simulink model "GlobalMessageLevel_R2010b"  (Simulink 7.6)
settings: Solver=ode45  StartTime=0.0  StopTime=10.0  RelTol=1e-3
undefined symbols (not defined in the file): Carnot_density_Callbacks, Carnot_GlobalMessageLevel_Callbacks
settings Model: DEBUGGLOBALLEVEL=DEBUG  DEBUGMAXTOTALWARNINGS=inf  DEBUGMAXCONSECUTIVEWARNINGS=inf  DEBUGWRITETOFILE=0  DEBUGFILENAME='error.txt'  Creator=awohlfei  LastModifiedBy=awohlfei
settings OptimizationCC: ExpressionDepthLimit=128
settings DebuggingCC: FcnCallInpInsideContextMsg=Enable All
settings CodeAppCC: CustomSymbolStrType=$N$R$M_T

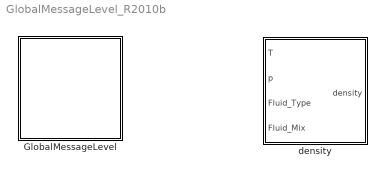
== system GlobalMessageLevel_R2010b ==
  GlobalMessageLevel : Subsystem  LoadFcn=Carnot_GlobalMessageLevel_Callbacks('LoadFcn');  mask(Global Message Level){GLOBALLOCAL=global, DEBUGLEVEL=DEBUG, MAXTOTALWARNINGS=inf, MAXCONSECUTIVEWARNINGS=inf, WRITETOFILE=0, FILENAME='error.txt'}
      mask prompts: GLOBALLOCAL "message settings"; DEBUGLEVEL "message level"; MAXTOTALWARNINGS "maximum total number of warnings"; MAXCONSECUTIVEWARNINGS "maxmum consecutive warnings"; WRITETOFILE "write messages to file"
      mask help: This block sets the message level of the complete model.
      mask init:
      | Carnot_GlobalMessageLevel_Callbacks('SetData');
      mask StyleString: popup(global|local),popup(DEBUG|INFO|WARNING|ERROR|FATAL|NONE),edit,edit,edit,edit
      mask CallbackString: Carnot_GlobalMessageLevel_Callbacks('MaskCallback');|||||
      mask Display:
      | fprintf(get_param(gcb, 'GLOBALLOCAL'));
      | fprintf(['\n\n', get_param(gcb, 'DEBUGLEVEL')]);
  density : Subsystem  LoadFcn=Carnot_density_Callbacks('LoadFcn');  InitFcn=load('THB.mat');  mask(density){INPUTARGUMENTS=state variables (classic), DEBUGLEVEL=DEBUG, MAXTOTALWARNINGS=inf, MAXCONSECUTIVEWARNINGS=inf, WRITETOFILE=0, FILENAME='errors.txt'}
      mask prompts: INPUTARGUMENTS "Input arguments"; DEBUGLEVEL "Debug level"; MAXTOTALWARNINGS "maximum number of total warning"; MAXCONSECUTIVEWARNINGS "maximum number of consecutive warnings"; WRITETOFILE "write messages to file"; FILENAME "filename for error messages"
      mask help:
      | Calculates the fluid density  [kg/m³].
      | Calls the function "density" in the CARNOT library "carlib".
      mask init:
      | %Inports
      | Carnot_density_Callbacks('CreateInports');
      | 
      | %global debug level
      | [DEBUGLEVEL, MAXTOTALWARNINGS, MAXCONSECUTIVEWARNINGS, WRITETOFILE, FILENAME] = Carnot_density_Callbacks('CheckDebugLevels', DEBUGLEVEL, MAXTOTALWARNINGS, MAXCONSECUTIVEWARNINGS, WRITETOFILE, FILENAME);
      mask StyleString: popup(state variables (classic)|THB|THV),popup(DEBUG|INFO|WARNING|ERROR|FATAL|NONE),edit,edit,edit,edit
      mask CallbackString: Carnot_density_Callbacks('MaskVisibilities');|||||
      mask TabNameString: Parameters,Debugging,Debugging,Debugging,Debugging,Debugging

== system GlobalMessageLevel_R2010b/GlobalMessageLevel ==

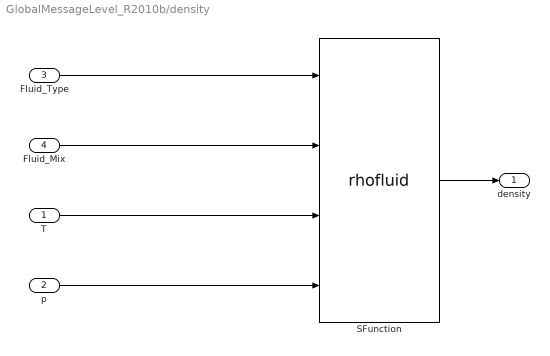
== system GlobalMessageLevel_R2010b/density ==
  T : Inport
  p : Inport  Port=2
  Fluid_Type : Inport  Port=3
  Fluid_Mix : Inport  Port=4
  SFunction : S-Function  FunctionName=rhofluid  Parameters=DEBUGLEVEL-1,MAXTOTALWARNINGS,MAXCONSECUTIVEWARNINGS,WRITETOFILE,FILENAME  EnableBusSupport=off
  density : Outport
  wires:
  SFunction/1 -> density/1
  T/1 -> SFunction/3
  p/1 -> SFunction/4
  Fluid_Type/1 -> SFunction/1
  Fluid_Mix/1 -> SFunction/2
